simulink model "vexv5_Vision_Monitor_Tune"  (R2019b)
settings: Solver=FixedStepAuto  StartTime=0.0  StopTime=inf  RelTol=1e-3
libraries: vexv5lib x1, simulink x1
settings Model: Creator=avenkata  LastModifiedBy=josea
settings OptimizationCC: EnhancedBackFolding=on  PassReuseOutputArgsThreshold=0  MaxStackSize=64  OptimizeBlockOrder=speed  DifferentSizesBufferReuse=on  OptimizationCustomize=off
settings DebuggingCC: ParameterTunabilityLossMsg=error  SymbolicDimsDataTypeCodeGenerationDiagnostic=none  ArithmeticOperatorsInVariantConditions=warning
settings HardwareCC: ProdBitPerPointer=32  ProdBitPerSizeT=32  ProdBitPerPtrDiffT=32  ProdLargestAtomicInteger=Long  ProdLargestAtomicFloat=Double  ProdWordSize=32  ProdHWDeviceType=ARM Compatible->ARM Cortex  UseEmbeddedCoderFeatures=off
settings SFSimCC: MATLABDynamicMemAlloc=off  CustomCodeUndefinedFunction=UseInterfaceOnly
settings RTWCC: SystemTargetFile=ert.tlc  HardwareBoard=VEX V5 Robot Brain  TLCOptions="-aInlineSetEventsForThisBaseRateFcn=TLC_FALSE -aSuppressMultiTaskScheduler=TLC_FALSE  -aRateBasedStepFcn=0"  TemplateMakefile=ert_default_tmf  GenerateReport=on  Toolchain=GNU Tools for ARM Embedded Processors  LaunchReport=on
settings CodeAppCC: ForceParamTrailComments=on  OperatorAnnotations=on
settings ERTTargetCC: ERTCustomFileBanners=off  SupportContinuousTime=on  SupportNonInlinedSFcns=on  RemoveResetFunc=off  ModelStepFunctionPrototypeControlCompliant=off

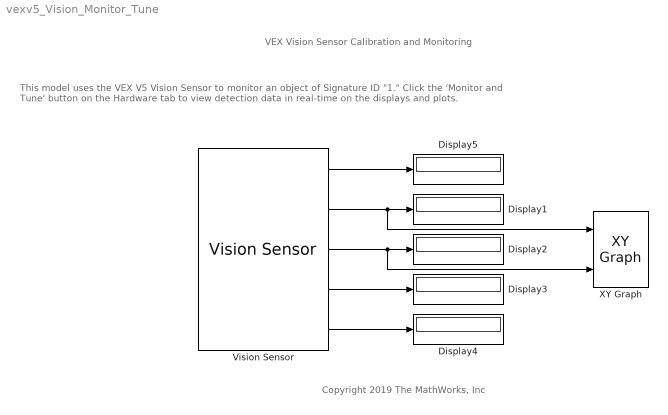
== system vexv5_Vision_Monitor_Tune ==
  note: This model uses the VEX V5 Vision Sensor to monitor an object of Signature ID "1."
      | Click the 'Monitor and Tune' button on the Hardware tab to view detection data in real-time on the displays and plots.
  note: VEX Vision Sensor
      | Calibration and Monitoring
  note: Copyright 2019 The MathWorks, Inc
  Display{1..5} (5 alike) : Display
  Vision Sensor : vexv5lib/Sensors/Vision Sensor  Port=5  EnableColorCode=off  ColorCode=12  SigId=SIG_1  size=1  LCDOutput=on  SampleTime=0.2
      settings: SourceProductName=Simulink Coder Support Package for VEX EDR V5 Robot Brain  SourceProductBaseCode=VEXV5
  XY Graph : simulink/Sinks/XY Graph  xmin=0  xmax=300  ymin=0  ymax=200  st=-1
  wires:
  Vision Sensor/1 -> Display5/1
  Vision Sensor/2 -> XY Graph/1, Display1/1
  Vision Sensor/3 -> XY Graph/2, Display2/1
  Vision Sensor/4 -> Display3/1
  Vision Sensor/5 -> Display4/1
